simulink model "SpdGovSwt_DD"  (R2016b)
settings: configuration reference "CodeGenConfigSet" (kept outside this file)
values from neighbouring files (symbols this model uses):
  SpdGovSwt_stDflVal_C = Calibration.Parameter    [init_SpdGovSwt_DD.m]    (also in init_SpdGovSwt_DD_SIL.m = Simulink.Parameter)
  SpdGovSwt_swtSigSel_C = Calibration.Parameter    [init_SpdGovSwt_DD.m]    (also in init_SpdGovSwt_DD_SIL.m = Simulink.Parameter)
  SpdGovSwt_tiDebHiLo_C = Calibration.Parameter    [init_SpdGovSwt_DD.m]    (also in init_SpdGovSwt_DD_SIL.m = Simulink.Parameter)
  SpdGovSwt_tiDebLoHi_C = Calibration.Parameter    [init_SpdGovSwt_DD.m]    (also in init_SpdGovSwt_DD_SIL.m = Simulink.Parameter)
undefined symbols (not defined in the file or in its folder): SpdGovSwt_DD_DT, Switch_conv
libraries: CXLib x1
settings Model: Creator=xinchangran  LastModifiedBy=xinchangran
settings ConfigSetRef: SourceLocation=Base Workspace

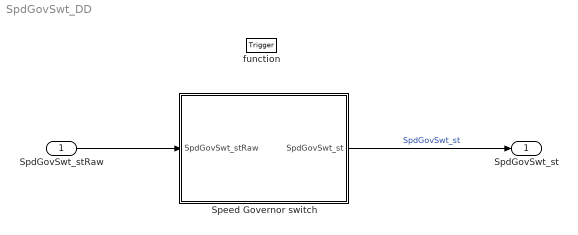
== system SpdGovSwt_DD ==
  SpdGovSwt_stRaw : Inport  Description=Speed Governor switch Raw  OutMin=0  OutMax=1  OutDataTypeStr=boolean
  function : TriggerPort  TriggerType=function-call  VariantControl=Variant
  Speed Governor switch : Subsystem
  SpdGovSwt_st : Outport  Description=Speed Governor Switch status  OutMin=0  OutMax=1  OutDataTypeStr=boolean
  wires:
  SpdGovSwt_stRaw/1 -> Speed Governor switch/1(SpdGovSwt_stRaw)
  Speed Governor switch/1(SpdGovSwt_st) -> SpdGovSwt_st/1  "SpdGovSwt_st"

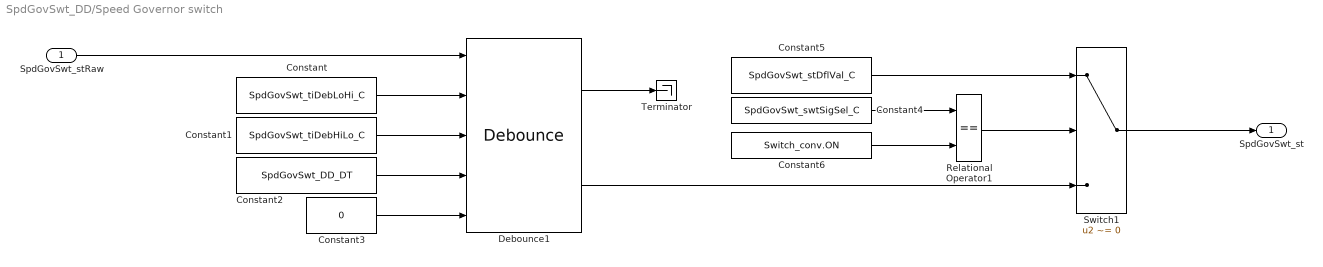
== system SpdGovSwt_DD/Speed Governor switch ==
  SpdGovSwt_stRaw : Inport
  Constant : Constant  Value=SpdGovSwt_tiDebLoHi_C
  Constant1 : Constant  Value=SpdGovSwt_tiDebHiLo_C
  Constant2 : Constant  Value=SpdGovSwt_DD_DT
  Constant3 : Constant  Value=0  OutDataTypeStr=Inherit: Inherit via back propagation
  Constant4 : Constant  Value=SpdGovSwt_swtSigSel_C
  Constant5 : Constant  Value=SpdGovSwt_stDflVal_C
  Constant6 : Constant  Value=Switch_conv.ON
  Debounce1 : CXLib/Debounce
  Relational Operator1 : RelationalOperator  Operator===  OutDataTypeStr=boolean  RndMeth=Nearest
  Switch1 : Switch  Criteria=u2 ~= 0
  Terminator : Terminator
  SpdGovSwt_st : Outport  Description=Speed Governor Switch status  OutMin=0  OutMax=1  OutDataTypeStr=boolean
  wires:
  Constant5/1 -> Switch1/1
  Debounce1/1 -> Terminator/1
  Constant1/1 -> Debounce1/3
  Constant2/1 -> Debounce1/4
  Constant3/1 -> Debounce1/5
  Constant/1 -> Debounce1/2
  Switch1/1 -> SpdGovSwt_st/1
  SpdGovSwt_stRaw/1 -> Debounce1/1
  Constant6/1 -> Relational Operator1/2
  Relational Operator1/1 -> Switch1/2
  Constant4/1 -> Relational Operator1/1
  Debounce1/2 -> Switch1/3
